simulink model "VFA_ActModel2_2015a"  (R2015a)
settings: Solver=ode23tb  SolverMode=SingleTasking  StartTime=tstart  StopTime=tsim  FixedStep=0.001  RelTol=1e-3
values from neighbouring files (symbols this model uses):
  Aa_M = zeros([10,10,length(TP.etasweep)])    [SimVFA.m]
  Ba32_aug_M = zeros([12,3,length(TP.etasweep)])    [SimVFA.m]
  Ba32_M = zeros([12,2,length(TP.etasweep)])    [SimVFA.m]
  Ba3_aug_M = zeros([12,3,length(TP.etasweep)])    [SimVFA.m]
  Ba3_M = zeros([12,2,length(TP.etasweep)])    [SimVFA.m]
  Ba_M = zeros([10,2,length(TP.etasweep)])    [SimVFA.m]
  Bp = TP.B_hold(:,1:5,SO.eta_nom+1)    [SimVFA.m]
  Ca = [C, zeros(size(C,1),length(index_output)) ... (first row only)    [SimVFA.m]
  Caz_M = zeros([2,10,length(TP.etasweep)])    [SimVFA.m]
  Cz = [0,0,0,0,1,0,0,0 ... (first row only)    [SimVFA.m]
  K_M = zeros([2,10,length(TP.etasweep)])    [SimVFA.m]
  L_M = zeros([10,3,length(TP.etasweep)])    [SimVFA.m]
  Rinv_M = zeros([3,3,length(TP.etasweep)])    [SimVFA.m]
  S1_M = zeros([2,3,length(TP.etasweep)])    [SimVFA.m]
  S_M = zeros([3,3,length(TP.etasweep)])    [SimVFA.m]
undefined symbols (not defined in the file or in its folder): a20, a21, a22, Aact, Acmd, Ada_Flag, ahold, Bact, Bact_x, Baz, Bcmd, Cact, Cact_dot, Ccmd, Ccmd_dot, cmd_filter_0, d00, d10, d11, d20, d21, d22, d_sam, data, Gamma_l, Gamma_p1, Gamma_p2, Gamma_p3, Gamma_p31, Gamma_p31xm, Gamma_p32, Gamma_vl, i_input_sel, i_state_sel, initstate, input_hold, inputselect, lambda_0, Lambda_s, mu_lambda, mu_psi1, mu_psi2, mu_psi3, mu_psi31, mu_psi32, n_sam, psi1_0, psi2_0, psi31_0, psi31xm_0, psi32_0, psi3_0, samplet, Si1, Si3, state_hold, vlambda_0, xact_0, xm_0
libraries: simulink x9
(part 2 of 2)

== system VFA_ActModel2_2015a/Adaptive Control/Fxm_Calculation/Filter13 ==
  u1 : Inport
  u1dot : Inport  Port=2
  u2 : Inport  Port=3
  u2dot : Inport  Port=4
  Gain2 : Gain  Gain=d10
  Gain25 : Gain  Gain=d11
  Matrix Multiply2 : Product  Multiplication=Matrix(*)
  Matrix Multiply3 : Product  Multiplication=Matrix(*)
  Sum2 : Sum  Inputs=++|
  Out1 : Outport
  wires:
  Matrix Multiply2/1 -> Gain2/1
  Matrix Multiply3/1 -> Gain25/1
  Gain25/1 -> Sum2/1
  u1dot/1 -> Matrix Multiply3/1
  u2/1 -> Matrix Multiply3/2
  u1/1 -> Matrix Multiply2/1
  u2dot/1 -> Matrix Multiply2/2
  Gain2/1 -> Sum2/2
  Sum2/1 -> Out1/1

== system VFA_ActModel2_2015a/Adaptive Control/Fxm_Calculation/Filter2 ==
  u1 : Inport
  u1dot : Inport  Port=2
  u2 : Inport  Port=3
  u2dot : Inport  Port=4
  Gain2 : Gain  Gain=d10
  Gain25 : Gain  Gain=d11
  Matrix Multiply2 : Product  Multiplication=Matrix(*)
  Matrix Multiply3 : Product  Multiplication=Matrix(*)
  Sum2 : Sum  Inputs=++|
  Out1 : Outport
  wires:
  Matrix Multiply2/1 -> Gain2/1
  Matrix Multiply3/1 -> Gain25/1
  Gain25/1 -> Sum2/1
  u1dot/1 -> Matrix Multiply3/1
  u2/1 -> Matrix Multiply3/2
  u1/1 -> Matrix Multiply2/1
  u2dot/1 -> Matrix Multiply2/2
  Gain2/1 -> Sum2/2
  Sum2/1 -> Out1/1

== system VFA_ActModel2_2015a/Adaptive Control/Fxm_Calculation/Filter3 ==
  u1 : Inport
  u1dot : Inport  Port=2
  u1ddot : Inport  Port=3
  u2 : Inport  Port=4
  u2dot : Inport  Port=5
  u2ddot : Inport  Port=6
  eta : Inport  Port=7
  Ba3 Interpolation : Subsystem
  Filter1 : Subsystem
      mask Display: disp('pi22 Mixer')
  Out1 : Outport
  wires:
  u2/1 -> Filter1/4(u2)
  u1/1 -> Filter1/1(u1)
  u1dot/1 -> Filter1/2(u1dot)
  u1ddot/1 -> Filter1/3(u1ddot)
  u2dot/1 -> Filter1/5(u2dot)
  u2ddot/1 -> Filter1/6(u2ddot)
  Filter1/1(Out1) -> Ba3 Interpolation/1(State)
  Ba3 Interpolation/1(Out1) -> Out1/1
  eta/1 -> Ba3 Interpolation/2(eta)

== system VFA_ActModel2_2015a/Adaptive Control/Fxm_Calculation/Filter4 ==
  In1 : Inport
  Add : Sum  Inputs=+--
  Add1 : Sum
  Add2 : Sum
  Gain1 : Gain  Gain=a21/a22
  Gain10 : Gain  Gain=1/a22
  Gain2 : Gain  Gain=a20/a22
  Gain3 : Gain  Gain=a21
  Gain4 : Gain  Gain=a21
  Gain{5..9} (5 alike) : Gain  Gain=a22
  Integrator : Integrator
  Integrator1 : Integrator
  pi20 filter : Outport
  pi20 filter dot : Outport  Port=2
  pi20 filter ddot : Outport  Port=3
  pi21 filter : Outport  Port=4
  pi21 filter dot : Outport  Port=5
  wires:
  Integrator/1 -> Gain1/1, Gain6/1, Integrator1/1, Gain4/1, Gain9/1  "out_dot"
  Add/1 -> Integrator/1, Gain8/1, Gain7/1  "out_ddot"
  Gain1/1 -> Add/3
  Gain2/1 -> Add/2
  Integrator1/1 -> Gain5/1, Gain3/1, Gain2/1  "out"
  Add1/1 -> pi21 filter/1
  Gain3/1 -> Add1/1
  Gain4/1 -> Add2/1
  Add2/1 -> pi21 filter dot/1
  Gain5/1 -> pi20 filter/1
  Gain6/1 -> pi20 filter dot/1
  Gain7/1 -> pi20 filter ddot/1
  Gain8/1 -> Add2/2
  Gain9/1 -> Add1/2
  In1/1 -> Gain10/1
  Gain10/1 -> Add/1

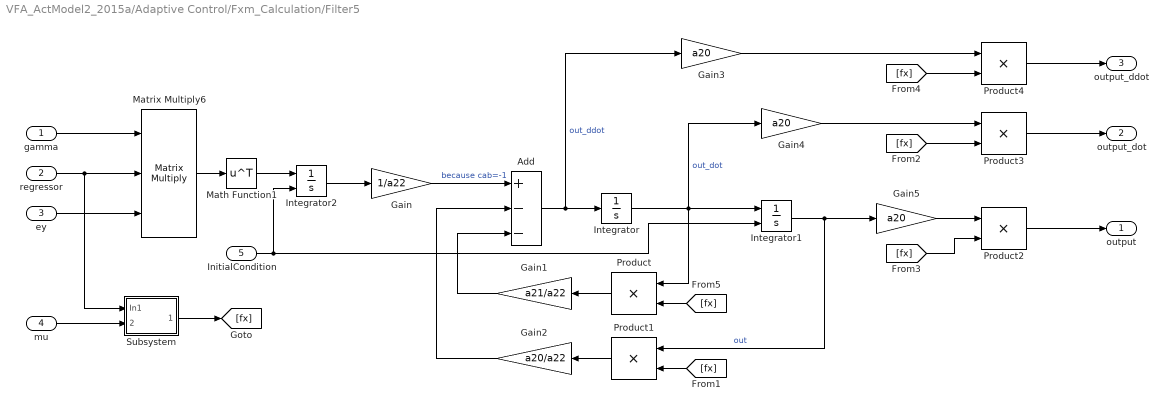
== system VFA_ActModel2_2015a/Adaptive Control/Fxm_Calculation/Filter5 ==
  gamma : Inport
  regressor : Inport  Port=2
  ey : Inport  Port=3
  mu : Inport  Port=4
  InitialCondition : Inport  Port=5
  Add : Sum  Inputs=+--
  Gain : Gain  Gain=1/a22
  Gain1 : Gain  Gain=a21/a22
  Gain2 : Gain  Gain=a20/a22
  Gain3 : Gain  Gain=a20
  Gain4 : Gain  Gain=a20
  Gain5 : Gain  Gain=a20
  Integrator : Integrator
  Integrator1 : Integrator  InitialConditionSource=external  InitialCondition=lambda_0'
  Integrator2 : Integrator  InitialConditionSource=external  InitialCondition=lambda_0'
  Math Function1 : Math  Operator=transpose  SaturateOnIntegerOverflow=on
  Matrix Multiply6 : Product  Inputs=3  Multiplication=Matrix(*)
  Product{,1..4} (5 alike) : Product  RndMeth=Zero
  Subsystem : Subsystem
      mask Display: disp('f(x)');
  output : Outport
  output_dot : Outport  Port=2
  output_ddot : Outport  Port=3
  wires:
  Integrator/1 -> Product/1, Gain4/1, Integrator1/1  "out_dot"
  Add/1 -> Integrator/1, Gain3/1  "out_ddot"
  Gain/1 -> Add/1  "because cab=-1"
  Gain1/1 -> Add/3
  Gain2/1 -> Add/2
  Integrator1/1 -> Product1/1, Gain5/1  "out"
  gamma/1 -> Matrix Multiply6/1
  regressor/1 -> Subsystem/1(In1), Matrix Multiply6/2
  ey/1 -> Matrix Multiply6/3
  Subsystem/1(Out1) -> [fx]
  Product/1 -> Gain1/1
  [fx] -> Product/2
  Product1/1 -> Gain2/1
  [fx] -> Product1/2
  Integrator2/1 -> Gain/1
  Gain5/1 -> Product2/1
  [fx] -> Product2/2
  Product2/1 -> output/1
  Gain4/1 -> Product3/1
  Product3/1 -> output_dot/1
  [fx] -> Product3/2
  [fx] -> Product4/2
  Gain3/1 -> Product4/1
  Product4/1 -> output_ddot/1
  Matrix Multiply6/1 -> Math Function1/1
  Math Function1/1 -> Integrator2/1
  InitialCondition/1 -> Integrator2/2, Integrator1/2
  mu/1 -> Subsystem/2(mu_psi)

== system VFA_ActModel2_2015a/Adaptive Control/Rinv and S Interpolation/Subsystem1 ==
  In1 : Inport
  In2 : Inport  Port=2
  Bias1 : Bias  Bias=1
  Direct Lookup Table (n-D)2 : LookupNDDirect  NumberOfTableDimensions=3  InputsSelectThisObjectFromTable=2-D Matrix  TableIsInput=on  Table=ahold
  Direct Lookup Table (n-D)3 : LookupNDDirect  NumberOfTableDimensions=3  InputsSelectThisObjectFromTable=2-D Matrix  TableIsInput=on  Table=ahold
  Fcn1 : Fcn  Expr=1-u(1)
  Prelookup1 : PreLookup  BreakpointsData=etasweep  ExtrapMethod=Linear
  Product2 : Product  RndMeth=Zero
  Product3 : Product  RndMeth=Zero
  Sum1 : Sum  Inputs=|++
  Out1 : Outport
  wires:
  In1/1 -> Prelookup1/1
  Sum1/1 -> Out1/1
  Prelookup1/1 -> Direct Lookup Table (n-D)3/1, Bias1/1
  Direct Lookup Table (n-D)2/1 -> Product2/1
  Prelookup1/2 -> Product2/2, Fcn1/1
  Direct Lookup Table (n-D)3/1 -> Product3/1
  Product2/1 -> Sum1/1
  Product3/1 -> Sum1/2
  Bias1/1 -> Direct Lookup Table (n-D)2/1
  In2/1 -> Direct Lookup Table (n-D)3/2, Direct Lookup Table (n-D)2/2
  Fcn1/1 -> Product3/2

== system VFA_ActModel2_2015a/Adaptive Control/Rinv and S Interpolation/Subsystem2 ==
  In1 : Inport
  In2 : Inport  Port=2
  Bias1 : Bias  Bias=1
  Direct Lookup Table (n-D)2 : LookupNDDirect  NumberOfTableDimensions=3  InputsSelectThisObjectFromTable=2-D Matrix  TableIsInput=on  Table=ahold
  Direct Lookup Table (n-D)3 : LookupNDDirect  NumberOfTableDimensions=3  InputsSelectThisObjectFromTable=2-D Matrix  TableIsInput=on  Table=ahold
  Fcn1 : Fcn  Expr=1-u(1)
  Prelookup1 : PreLookup  BreakpointsData=etasweep  ExtrapMethod=Linear
  Product2 : Product  RndMeth=Zero
  Product3 : Product  RndMeth=Zero
  Sum1 : Sum  Inputs=|++
  Out1 : Outport
  wires:
  In1/1 -> Prelookup1/1
  Sum1/1 -> Out1/1
  Prelookup1/1 -> Direct Lookup Table (n-D)3/1, Bias1/1
  Direct Lookup Table (n-D)2/1 -> Product2/1
  Prelookup1/2 -> Product2/2, Fcn1/1
  Direct Lookup Table (n-D)3/1 -> Product3/1
  Product2/1 -> Sum1/1
  Product3/1 -> Sum1/2
  Bias1/1 -> Direct Lookup Table (n-D)2/1
  In2/1 -> Direct Lookup Table (n-D)3/2, Direct Lookup Table (n-D)2/2
  Fcn1/1 -> Product3/2

== system VFA_ActModel2_2015a/Adaptive Control/S Interpolation/Subsystem1 ==
  In1 : Inport
  In2 : Inport  Port=2
  Bias1 : Bias  Bias=1
  Direct Lookup Table (n-D)2 : LookupNDDirect  NumberOfTableDimensions=3  InputsSelectThisObjectFromTable=2-D Matrix  TableIsInput=on  Table=ahold
  Direct Lookup Table (n-D)3 : LookupNDDirect  NumberOfTableDimensions=3  InputsSelectThisObjectFromTable=2-D Matrix  TableIsInput=on  Table=ahold
  Fcn1 : Fcn  Expr=1-u(1)
  Prelookup1 : PreLookup  BreakpointsData=etasweep  ExtrapMethod=Linear
  Product2 : Product  RndMeth=Zero
  Product3 : Product  RndMeth=Zero
  Sum1 : Sum  Inputs=|++
  Out1 : Outport
  wires:
  In1/1 -> Prelookup1/1
  Sum1/1 -> Out1/1
  Prelookup1/1 -> Direct Lookup Table (n-D)3/1, Bias1/1
  Direct Lookup Table (n-D)2/1 -> Product2/1
  Prelookup1/2 -> Product2/2, Fcn1/1
  Direct Lookup Table (n-D)3/1 -> Product3/1
  Product2/1 -> Sum1/1
  Product3/1 -> Sum1/2
  Bias1/1 -> Direct Lookup Table (n-D)2/1
  In2/1 -> Direct Lookup Table (n-D)3/2, Direct Lookup Table (n-D)2/2
  Fcn1/1 -> Product3/2

== system VFA_ActModel2_2015a/Adaptive Control/S1 Interpolation/Subsystem1 ==
  In1 : Inport
  In2 : Inport  Port=2
  Bias1 : Bias  Bias=1
  Direct Lookup Table (n-D)2 : LookupNDDirect  NumberOfTableDimensions=3  InputsSelectThisObjectFromTable=2-D Matrix  TableIsInput=on  Table=ahold
  Direct Lookup Table (n-D)3 : LookupNDDirect  NumberOfTableDimensions=3  InputsSelectThisObjectFromTable=2-D Matrix  TableIsInput=on  Table=ahold
  Fcn1 : Fcn  Expr=1-u(1)
  Prelookup1 : PreLookup  BreakpointsData=etasweep  ExtrapMethod=Linear
  Product2 : Product  RndMeth=Zero
  Product3 : Product  RndMeth=Zero
  Sum1 : Sum  Inputs=|++
  Out1 : Outport
  wires:
  In1/1 -> Prelookup1/1
  Sum1/1 -> Out1/1
  Prelookup1/1 -> Direct Lookup Table (n-D)3/1, Bias1/1
  Direct Lookup Table (n-D)2/1 -> Product2/1
  Prelookup1/2 -> Product2/2, Fcn1/1
  Direct Lookup Table (n-D)3/1 -> Product3/1
  Product2/1 -> Sum1/1
  Product3/1 -> Sum1/2
  Bias1/1 -> Direct Lookup Table (n-D)2/1
  In2/1 -> Direct Lookup Table (n-D)3/2, Direct Lookup Table (n-D)2/2
  Fcn1/1 -> Product3/2

== system VFA_ActModel2_2015a/Adaptive Control/uad_Calculation/Filter1 ==
  u1 : Inport
  u1dot : Inport  Port=2
  u1ddot : Inport  Port=3
  u2 : Inport  Port=4
  u2dot : Inport  Port=5
  u2ddot : Inport  Port=6
  Gain1 : Gain  Gain=d21
  Gain2 : Gain  Gain=d20
  Gain3 : Gain  Gain=d22
  Gain4 : Gain  Gain=a22
  Gain5 : Gain  Gain=d11
  Gain6 : Gain  Gain=d10
  Gain7 : Gain  Gain=a21
  Gain8 : Gain  Gain=d00
  Gain9 : Gain  Gain=a20
  Matrix Multiply{1..6} (6 alike) : Product  Multiplication=Matrix(*)
  Sum1 : Sum  Inputs=+++|
  Sum2 : Sum  Inputs=+++|
  Sum3 : Sum  Inputs=++|
  Out1 : Outport
  wires:
  u1/1 -> Matrix Multiply2/1, Matrix Multiply6/1, Matrix Multiply5/1
  u2ddot/1 -> Matrix Multiply2/2
  Matrix Multiply2/1 -> Gain2/1
  u1ddot/1 -> Matrix Multiply1/1
  u2/1 -> Matrix Multiply6/2, Matrix Multiply4/2, Matrix Multiply1/2
  Matrix Multiply1/1 -> Gain3/1
  u2dot/1 -> Matrix Multiply5/2, Matrix Multiply3/2
  u1dot/1 -> Matrix Multiply4/1, Matrix Multiply3/1
  Matrix Multiply3/1 -> Gain1/1
  Gain1/1 -> Sum1/3
  Gain3/1 -> Sum1/2
  Gain2/1 -> Sum1/1
  Sum1/1 -> Gain4/1
  Gain4/1 -> Sum2/1
  Matrix Multiply4/1 -> Gain5/1
  Gain5/1 -> Sum3/1
  Matrix Multiply5/1 -> Gain6/1
  Gain6/1 -> Sum3/2
  Sum3/1 -> Gain7/1
  Gain7/1 -> Sum2/2
  Matrix Multiply6/1 -> Gain8/1
  Gain8/1 -> Gain9/1
  Sum2/1 -> Out1/1
  Gain9/1 -> Sum2/3

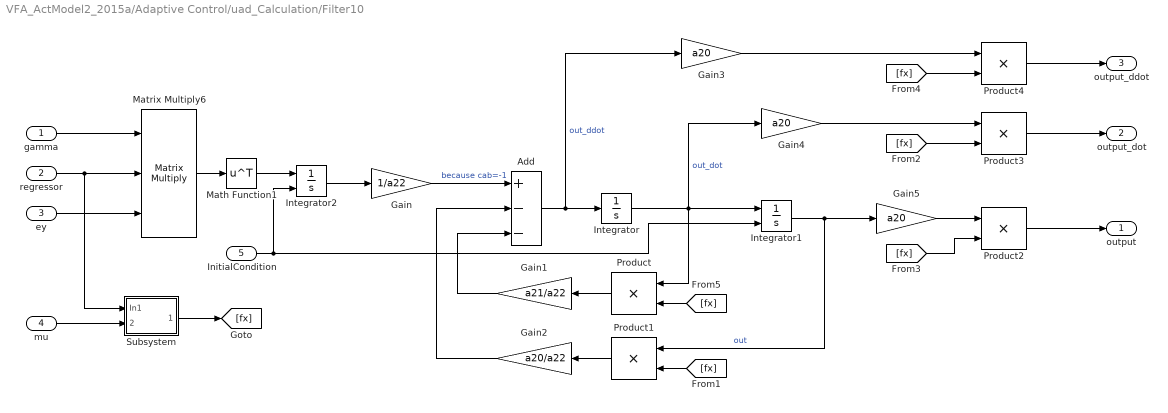
== system VFA_ActModel2_2015a/Adaptive Control/uad_Calculation/Filter10 ==
  gamma : Inport
  regressor : Inport  Port=2
  ey : Inport  Port=3
  mu : Inport  Port=4
  InitialCondition : Inport  Port=5
  Add : Sum  Inputs=+--
  Gain : Gain  Gain=1/a22
  Gain1 : Gain  Gain=a21/a22
  Gain2 : Gain  Gain=a20/a22
  Gain3 : Gain  Gain=a20
  Gain4 : Gain  Gain=a20
  Gain5 : Gain  Gain=a20
  Integrator : Integrator
  Integrator1 : Integrator  InitialConditionSource=external  InitialCondition=lambda_0'
  Integrator2 : Integrator  InitialConditionSource=external  InitialCondition=lambda_0'
  Math Function1 : Math  Operator=transpose  SaturateOnIntegerOverflow=on
  Matrix Multiply6 : Product  Inputs=3  Multiplication=Matrix(*)
  Product{,1..4} (5 alike) : Product  RndMeth=Zero
  Subsystem : Subsystem
      mask Display: disp('f(x)');
  output : Outport
  output_dot : Outport  Port=2
  output_ddot : Outport  Port=3
  wires:
  Integrator/1 -> Product/1, Gain4/1, Integrator1/1  "out_dot"
  Add/1 -> Integrator/1, Gain3/1  "out_ddot"
  Gain/1 -> Add/1  "because cab=-1"
  Gain1/1 -> Add/3
  Gain2/1 -> Add/2
  Integrator1/1 -> Product1/1, Gain5/1  "out"
  gamma/1 -> Matrix Multiply6/1
  regressor/1 -> Subsystem/1(In1), Matrix Multiply6/2
  ey/1 -> Matrix Multiply6/3
  Subsystem/1(Out1) -> [fx]
  Product/1 -> Gain1/1
  [fx] -> Product/2
  Product1/1 -> Gain2/1
  [fx] -> Product1/2
  Integrator2/1 -> Gain/1
  Gain5/1 -> Product2/1
  [fx] -> Product2/2
  Product2/1 -> output/1
  Gain4/1 -> Product3/1
  Product3/1 -> output_dot/1
  [fx] -> Product3/2
  [fx] -> Product4/2
  Gain3/1 -> Product4/1
  Product4/1 -> output_ddot/1
  Matrix Multiply6/1 -> Math Function1/1
  Math Function1/1 -> Integrator2/1
  InitialCondition/1 -> Integrator2/2, Integrator1/2
  mu/1 -> Subsystem/2(mu_psi)

== system VFA_ActModel2_2015a/Adaptive Control/uad_Calculation/Filter11 ==
  u1 : Inport
  u1dot : Inport  Port=2
  u1ddot : Inport  Port=3
  u2 : Inport  Port=4
  u2dot : Inport  Port=5
  u2ddot : Inport  Port=6
  Gain1 : Gain  Gain=d21
  Gain2 : Gain  Gain=d20
  Gain3 : Gain  Gain=d22
  Gain4 : Gain  Gain=a22
  Gain5 : Gain  Gain=d11
  Gain6 : Gain  Gain=d10
  Gain7 : Gain  Gain=a21
  Gain8 : Gain  Gain=d00
  Gain9 : Gain  Gain=a20
  Matrix Multiply{1..6} (6 alike) : Product  Multiplication=Matrix(*)
  Sum1 : Sum  Inputs=+++|
  Sum2 : Sum  Inputs=+++|
  Sum3 : Sum  Inputs=++|
  Out1 : Outport
  wires:
  u1/1 -> Matrix Multiply2/1, Matrix Multiply6/1, Matrix Multiply5/1
  u2ddot/1 -> Matrix Multiply2/2
  Matrix Multiply2/1 -> Gain2/1
  u1ddot/1 -> Matrix Multiply1/1
  u2/1 -> Matrix Multiply6/2, Matrix Multiply4/2, Matrix Multiply1/2
  Matrix Multiply1/1 -> Gain3/1
  u2dot/1 -> Matrix Multiply5/2, Matrix Multiply3/2
  u1dot/1 -> Matrix Multiply4/1, Matrix Multiply3/1
  Matrix Multiply3/1 -> Gain1/1
  Gain1/1 -> Sum1/3
  Gain3/1 -> Sum1/2
  Gain2/1 -> Sum1/1
  Sum1/1 -> Gain4/1
  Gain4/1 -> Sum2/1
  Matrix Multiply4/1 -> Gain5/1
  Gain5/1 -> Sum3/1
  Matrix Multiply5/1 -> Gain6/1
  Gain6/1 -> Sum3/2
  Sum3/1 -> Gain7/1
  Gain7/1 -> Sum2/2
  Matrix Multiply6/1 -> Gain8/1
  Gain8/1 -> Gain9/1
  Sum2/1 -> Out1/1
  Gain9/1 -> Sum2/3

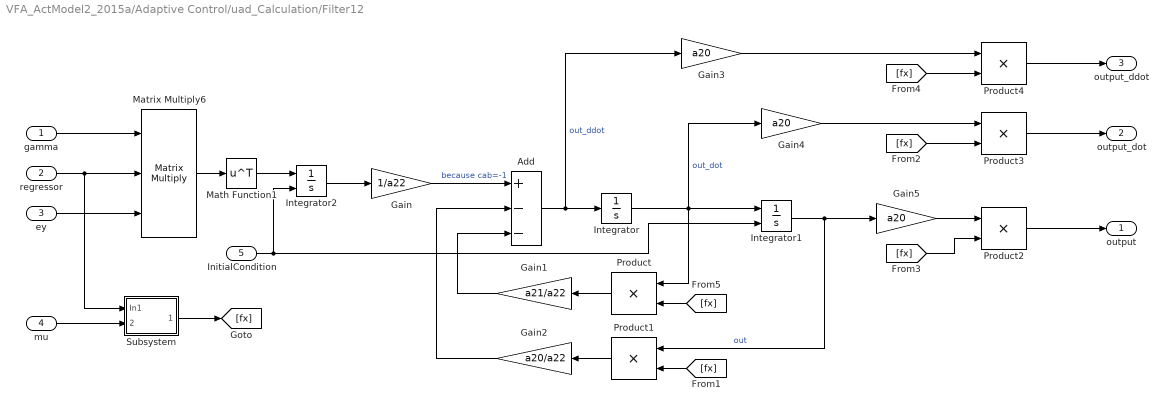
== system VFA_ActModel2_2015a/Adaptive Control/uad_Calculation/Filter12 ==
  gamma : Inport
  regressor : Inport  Port=2
  ey : Inport  Port=3
  mu : Inport  Port=4
  InitialCondition : Inport  Port=5
  Add : Sum  Inputs=+--
  Gain : Gain  Gain=1/a22
  Gain1 : Gain  Gain=a21/a22
  Gain2 : Gain  Gain=a20/a22
  Gain3 : Gain  Gain=a20
  Gain4 : Gain  Gain=a20
  Gain5 : Gain  Gain=a20
  Integrator : Integrator
  Integrator1 : Integrator  InitialConditionSource=external  InitialCondition=lambda_0'
  Integrator2 : Integrator  InitialConditionSource=external  InitialCondition=lambda_0'
  Math Function1 : Math  Operator=transpose  SaturateOnIntegerOverflow=on
  Matrix Multiply6 : Product  Inputs=3  Multiplication=Matrix(*)
  Product{,1..4} (5 alike) : Product  RndMeth=Zero
  Subsystem : Subsystem
      mask Display: disp('f(x)');
  output : Outport
  output_dot : Outport  Port=2
  output_ddot : Outport  Port=3
  wires:
  Integrator/1 -> Product/1, Gain4/1, Integrator1/1  "out_dot"
  Add/1 -> Integrator/1, Gain3/1  "out_ddot"
  Gain/1 -> Add/1  "because cab=-1"
  Gain1/1 -> Add/3
  Gain2/1 -> Add/2
  Integrator1/1 -> Product1/1, Gain5/1  "out"
  gamma/1 -> Matrix Multiply6/1
  regressor/1 -> Subsystem/1(In1), Matrix Multiply6/2
  ey/1 -> Matrix Multiply6/3
  Subsystem/1(Out1) -> [fx]
  Product/1 -> Gain1/1
  [fx] -> Product/2
  Product1/1 -> Gain2/1
  [fx] -> Product1/2
  Integrator2/1 -> Gain/1
  Gain5/1 -> Product2/1
  [fx] -> Product2/2
  Product2/1 -> output/1
  Gain4/1 -> Product3/1
  Product3/1 -> output_dot/1
  [fx] -> Product3/2
  [fx] -> Product4/2
  Gain3/1 -> Product4/1
  Product4/1 -> output_ddot/1
  Matrix Multiply6/1 -> Math Function1/1
  Math Function1/1 -> Integrator2/1
  InitialCondition/1 -> Integrator2/2, Integrator1/2
  mu/1 -> Subsystem/2(mu_psi)

== system VFA_ActModel2_2015a/Adaptive Control/uad_Calculation/Filter13 ==
  In1 : Inport
  In1_dot : Inport  Port=2
  Add : Sum  Inputs=+--
  Add1 : Sum
  Add2 : Sum
  Add3 : Sum  Inputs=-+
  Gain1 : Gain  Gain=a21/a22
  Gain10 : Gain  Gain=1/a22
  Gain11 : Gain  Gain=a20
  Gain2 : Gain  Gain=a20/a22
  Gain3 : Gain  Gain=a21
  Gain4 : Gain  Gain=a21
  Gain{5..9} (5 alike) : Gain  Gain=a22
  Integrator : Integrator
  Integrator1 : Integrator
  pi20 filter : Outport
  pi20 filter dot : Outport  Port=2
  pi20 filter ddot : Outport  Port=3
  pi21 filter : Outport  Port=4
  pi21 filter dot : Outport  Port=5
  pi21 filter ddot : Outport  Port=6
  wires:
  Integrator/1 -> Gain1/1, Gain11/1, Gain4/1, Gain9/1, Integrator1/1, Gain6/1  "out_dot"
  Add/1 -> Integrator/1, Gain8/1, Gain7/1  "out_ddot"
  Gain1/1 -> Add/3
  Gain2/1 -> Add/2
  Integrator1/1 -> Gain5/1, Gain3/1, Gain2/1  "out"
  Add1/1 -> pi21 filter/1
  Gain3/1 -> Add1/1
  Gain4/1 -> Add2/1
  Add2/1 -> pi21 filter dot/1
  Gain5/1 -> pi20 filter/1
  Gain6/1 -> pi20 filter dot/1
  Gain7/1 -> pi20 filter ddot/1
  Gain8/1 -> Add2/2
  Gain9/1 -> Add1/2
  In1/1 -> Gain10/1
  Gain10/1 -> Add/1
  Add3/1 -> pi21 filter ddot/1
  In1_dot/1 -> Add3/2
  Gain11/1 -> Add3/1

== system VFA_ActModel2_2015a/Adaptive Control/uad_Calculation/Filter2 ==
  u1 : Inport
  u1dot : Inport  Port=2
  u1ddot : Inport  Port=3
  u2 : Inport  Port=4
  u2dot : Inport  Port=5
  u2ddot : Inport  Port=6
  Gain1 : Gain  Gain=d21
  Gain2 : Gain  Gain=d20
  Gain3 : Gain  Gain=d22
  Gain4 : Gain  Gain=a22
  Gain5 : Gain  Gain=d11
  Gain6 : Gain  Gain=d10
  Gain7 : Gain  Gain=a21
  Gain8 : Gain  Gain=d00
  Gain9 : Gain  Gain=a20
  Matrix Multiply{1..6} (6 alike) : Product  Multiplication=Matrix(*)
  Sum1 : Sum  Inputs=+++|
  Sum2 : Sum  Inputs=+++|
  Sum3 : Sum  Inputs=++|
  Out1 : Outport
  wires:
  u1/1 -> Matrix Multiply2/1, Matrix Multiply6/1, Matrix Multiply5/1
  u2ddot/1 -> Matrix Multiply2/2
  Matrix Multiply2/1 -> Gain2/1
  u1ddot/1 -> Matrix Multiply1/1
  u2/1 -> Matrix Multiply6/2, Matrix Multiply4/2, Matrix Multiply1/2
  Matrix Multiply1/1 -> Gain3/1
  u2dot/1 -> Matrix Multiply5/2, Matrix Multiply3/2
  u1dot/1 -> Matrix Multiply4/1, Matrix Multiply3/1
  Matrix Multiply3/1 -> Gain1/1
  Gain1/1 -> Sum1/3
  Gain3/1 -> Sum1/2
  Gain2/1 -> Sum1/1
  Sum1/1 -> Gain4/1
  Gain4/1 -> Sum2/1
  Matrix Multiply4/1 -> Gain5/1
  Gain5/1 -> Sum3/1
  Matrix Multiply5/1 -> Gain6/1
  Gain6/1 -> Sum3/2
  Sum3/1 -> Gain7/1
  Gain7/1 -> Sum2/2
  Matrix Multiply6/1 -> Gain8/1
  Gain8/1 -> Gain9/1
  Sum2/1 -> Out1/1
  Gain9/1 -> Sum2/3

== system VFA_ActModel2_2015a/Adaptive Control/uad_Calculation/Filter3 ==
  u1 : Inport
  u1dot : Inport  Port=2
  u1ddot : Inport  Port=3
  u2 : Inport  Port=4
  u2dot : Inport  Port=5
  u2ddot : Inport  Port=6
  Gain1 : Gain  Gain=d21
  Gain2 : Gain  Gain=d20
  Gain3 : Gain  Gain=d22
  Gain4 : Gain  Gain=a22
  Gain5 : Gain  Gain=d11
  Gain6 : Gain  Gain=d10
  Gain7 : Gain  Gain=a21
  Gain8 : Gain  Gain=d00
  Gain9 : Gain  Gain=a20
  Matrix Multiply{1..6} (6 alike) : Product  Multiplication=Matrix(*)
  Sum1 : Sum  Inputs=+++|
  Sum2 : Sum  Inputs=+++|
  Sum3 : Sum  Inputs=++|
  Out1 : Outport
  wires:
  u1/1 -> Matrix Multiply2/1, Matrix Multiply6/1, Matrix Multiply5/1
  u2ddot/1 -> Matrix Multiply2/2
  Matrix Multiply2/1 -> Gain2/1
  u1ddot/1 -> Matrix Multiply1/1
  u2/1 -> Matrix Multiply6/2, Matrix Multiply4/2, Matrix Multiply1/2
  Matrix Multiply1/1 -> Gain3/1
  u2dot/1 -> Matrix Multiply5/2, Matrix Multiply3/2
  u1dot/1 -> Matrix Multiply4/1, Matrix Multiply3/1
  Matrix Multiply3/1 -> Gain1/1
  Gain1/1 -> Sum1/3
  Gain3/1 -> Sum1/2
  Gain2/1 -> Sum1/1
  Sum1/1 -> Gain4/1
  Gain4/1 -> Sum2/1
  Matrix Multiply4/1 -> Gain5/1
  Gain5/1 -> Sum3/1
  Matrix Multiply5/1 -> Gain6/1
  Gain6/1 -> Sum3/2
  Sum3/1 -> Gain7/1
  Gain7/1 -> Sum2/2
  Matrix Multiply6/1 -> Gain8/1
  Gain8/1 -> Gain9/1
  Sum2/1 -> Out1/1
  Gain9/1 -> Sum2/3

== system VFA_ActModel2_2015a/Adaptive Control/uad_Calculation/Filter4 ==
  note: out_ddot
  In1 : Inport
  Gain : Gain  Gain=1/a22
  Gain1 : Gain  Gain=a21/a22
  Gain2 : Gain  Gain=a20/a22
  Integrator : Integrator
  Integrator1 : Integrator
  Sum : Sum  Inputs=|+--
  Out1 : Outport
  Out2 : Outport  Port=2
  Out3 : Outport  Port=3
  wires:
  In1/1 -> Gain/1
  Gain/1 -> Sum/1
  Gain1/1 -> Sum/3
  Gain2/1 -> Sum/2
  Integrator1/1 -> Out1/1, Gain2/1  "out"
  Integrator/1 -> Gain1/1, Out2/1, Integrator1/1  "out_dot"
  Sum/1 -> Out3/1, Integrator/1

== system VFA_ActModel2_2015a/Adaptive Control/uad_Calculation/Filter5 ==
  xm : Inport
  r : Inport  Port=2
  r_dot : Inport  Port=3
  ey : Inport  Port=4
  Add : Sum  Inputs=2
  Add1 : Sum  Inputs=+++-
  Gain1 : Gain  Gain=Baz  Multiplication=Matrix(K*u)
  Gain2 : Gain  Gain=Baz  Multiplication=Matrix(K*u)
  Gain4 : Gain  Gain=Baz  Multiplication=Matrix(K*u)
  Matrix Multiply1 : Product  Inputs=3  Multiplication=Matrix(*)
  Matrix Multiply2 : Product  Multiplication=Matrix(*)
  Matrix Multiply3 : Product  Multiplication=Matrix(*)
  Matrix Multiply4 : Product  Inputs=3  Multiplication=Matrix(*)
  Out1 : Outport
  Out1_dot : Outport  Port=2
  Out1_ddot : Outport  Port=3
  wires:
  Matrix Multiply2/1 -> Add/1
  r/1 -> Gain2/1, Gain1/1
  r_dot/1 -> Gain4/1
  ey/1 -> Matrix Multiply4/3
  Add1/1 -> Out1_ddot/1  "(A^2)*xm + A*Bz*r + Bz*r_dot + A*L*ey"
  Gain1/1 -> Add/2
  Add/1 -> Out1_dot/1  "A*xm + Bz*r"
  Matrix Multiply1/1 -> Add1/1
  Matrix Multiply3/1 -> Add1/2
  Gain4/1 -> Add1/3
  Matrix Multiply4/1 -> Add1/4
  [Aa] -> Matrix Multiply2/1
  [Aa] -> Matrix Multiply1/1, Matrix Multiply1/2
  xm/1 -> Out1/1, Matrix Multiply1/3, Matrix Multiply2/2  "xm"
  [Aa] -> Matrix Multiply3/1
  [L] -> Matrix Multiply4/2
  [Aa] -> Matrix Multiply4/1
  Gain2/1 -> Matrix Multiply3/2

== system VFA_ActModel2_2015a/Adaptive Control/uad_Calculation/Filter6 ==
  In1 : Inport
  Integrator1 : Integrator
  Out1 : Outport
  Out1_dot : Outport  Port=2
  wires:
  Integrator1/1 -> Out1/1  "out"
  In1/1 -> Out1_dot/1, Integrator1/1

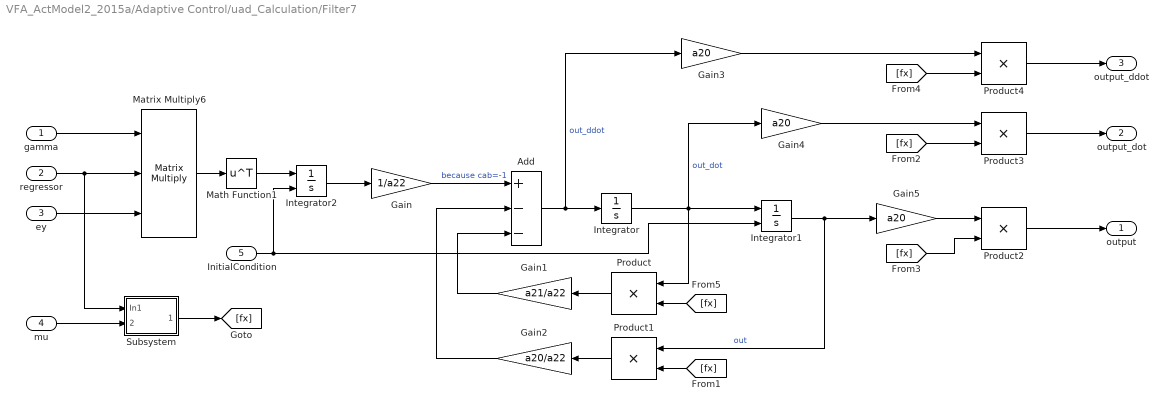
== system VFA_ActModel2_2015a/Adaptive Control/uad_Calculation/Filter7 ==
  gamma : Inport
  regressor : Inport  Port=2
  ey : Inport  Port=3
  mu : Inport  Port=4
  InitialCondition : Inport  Port=5
  Add : Sum  Inputs=+--
  Gain : Gain  Gain=1/a22
  Gain1 : Gain  Gain=a21/a22
  Gain2 : Gain  Gain=a20/a22
  Gain3 : Gain  Gain=a20
  Gain4 : Gain  Gain=a20
  Gain5 : Gain  Gain=a20
  Integrator : Integrator
  Integrator1 : Integrator  InitialConditionSource=external  InitialCondition=lambda_0'
  Integrator2 : Integrator  InitialConditionSource=external  InitialCondition=lambda_0'
  Math Function1 : Math  Operator=transpose  SaturateOnIntegerOverflow=on
  Matrix Multiply6 : Product  Inputs=3  Multiplication=Matrix(*)
  Product{,1..4} (5 alike) : Product  RndMeth=Zero
  Subsystem : Subsystem
      mask Display: disp('f(x)');
  output : Outport
  output_dot : Outport  Port=2
  output_ddot : Outport  Port=3
  wires:
  Integrator/1 -> Product/1, Gain4/1, Integrator1/1  "out_dot"
  Add/1 -> Integrator/1, Gain3/1  "out_ddot"
  Gain/1 -> Add/1  "because cab=-1"
  Gain1/1 -> Add/3
  Gain2/1 -> Add/2
  Integrator1/1 -> Product1/1, Gain5/1  "out"
  gamma/1 -> Matrix Multiply6/1
  regressor/1 -> Subsystem/1(In1), Matrix Multiply6/2
  ey/1 -> Matrix Multiply6/3
  Subsystem/1(Out1) -> [fx]
  Product/1 -> Gain1/1
  [fx] -> Product/2
  Product1/1 -> Gain2/1
  [fx] -> Product1/2
  Integrator2/1 -> Gain/1
  Gain5/1 -> Product2/1
  [fx] -> Product2/2
  Product2/1 -> output/1
  Gain4/1 -> Product3/1
  Product3/1 -> output_dot/1
  [fx] -> Product3/2
  [fx] -> Product4/2
  Gain3/1 -> Product4/1
  Product4/1 -> output_ddot/1
  Matrix Multiply6/1 -> Math Function1/1
  Math Function1/1 -> Integrator2/1
  InitialCondition/1 -> Integrator2/2, Integrator1/2
  mu/1 -> Subsystem/2(mu_psi)

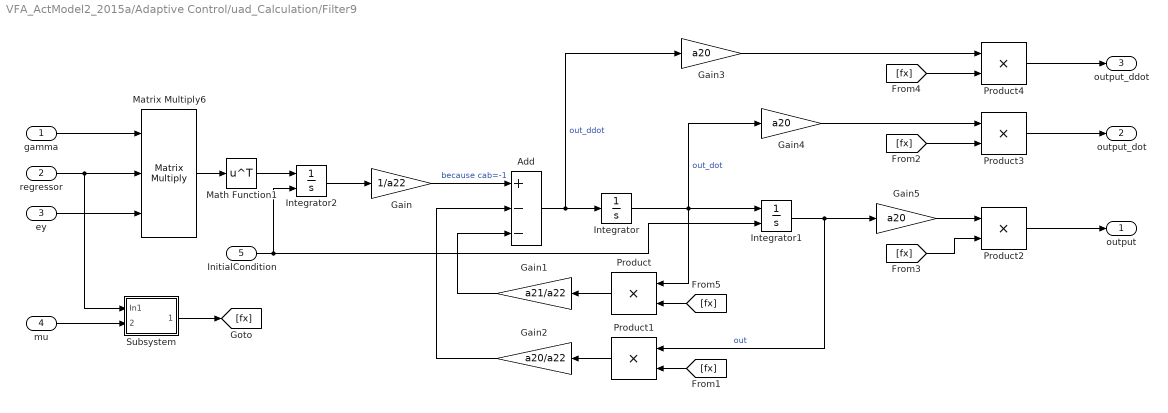
== system VFA_ActModel2_2015a/Adaptive Control/uad_Calculation/Filter9 ==
  gamma : Inport
  regressor : Inport  Port=2
  ey : Inport  Port=3
  mu : Inport  Port=4
  InitialCondition : Inport  Port=5
  Add : Sum  Inputs=+--
  Gain : Gain  Gain=1/a22
  Gain1 : Gain  Gain=a21/a22
  Gain2 : Gain  Gain=a20/a22
  Gain3 : Gain  Gain=a20
  Gain4 : Gain  Gain=a20
  Gain5 : Gain  Gain=a20
  Integrator : Integrator
  Integrator1 : Integrator  InitialConditionSource=external  InitialCondition=lambda_0'
  Integrator2 : Integrator  InitialConditionSource=external  InitialCondition=lambda_0'
  Math Function1 : Math  Operator=transpose  SaturateOnIntegerOverflow=on
  Matrix Multiply6 : Product  Inputs=3  Multiplication=Matrix(*)
  Product{,1..4} (5 alike) : Product  RndMeth=Zero
  Subsystem : Subsystem
      mask Display: disp('f(x)');
  output : Outport
  output_dot : Outport  Port=2
  output_ddot : Outport  Port=3
  wires:
  Integrator/1 -> Product/1, Gain4/1, Integrator1/1  "out_dot"
  Add/1 -> Integrator/1, Gain3/1  "out_ddot"
  Gain/1 -> Add/1  "because cab=-1"
  Gain1/1 -> Add/3
  Gain2/1 -> Add/2
  Integrator1/1 -> Product1/1, Gain5/1  "out"
  gamma/1 -> Matrix Multiply6/1
  regressor/1 -> Subsystem/1(In1), Matrix Multiply6/2
  ey/1 -> Matrix Multiply6/3
  Subsystem/1(Out1) -> [fx]
  Product/1 -> Gain1/1
  [fx] -> Product/2
  Product1/1 -> Gain2/1
  [fx] -> Product1/2
  Integrator2/1 -> Gain/1
  Gain5/1 -> Product2/1
  [fx] -> Product2/2
  Product2/1 -> output/1
  Gain4/1 -> Product3/1
  Product3/1 -> output_dot/1
  [fx] -> Product3/2
  [fx] -> Product4/2
  Gain3/1 -> Product4/1
  Product4/1 -> output_ddot/1
  Matrix Multiply6/1 -> Math Function1/1
  Math Function1/1 -> Integrator2/1
  InitialCondition/1 -> Integrator2/2, Integrator1/2
  mu/1 -> Subsystem/2(mu_psi)

== system VFA_ActModel2_2015a/Aircraft (Plant)/NonLinear VFA Model/Input Trim ==
  Constant1 : Constant  Value=[1:5]
  Constant2 : Constant  Value=input_hold
  Selector1 : Selector  InputPortWidth=9  IndexOptions=Index vector (port)  Indices=[1 3]  OutputSizes=1
  u_trim : Outport
  wires:
  Constant1/1 -> Selector1/2
  Constant2/1 -> Selector1/1
  Selector1/1 -> u_trim/1

== system VFA_ActModel2_2015a/Aircraft (Plant)/NonLinear VFA Model/State Trim ==
  Constant3 : Constant  Value=state_hold
  Constant5 : Constant  Value=i_state_sel
  Selector2 : Selector  InputPortWidth=length(Bp)  IndexOptions=Index vector (port)  Indices=[1 3]  OutputSizes=1
  To Workspace3 : ToWorkspace  VariableName=x_hold  SampleTime=-1
      settings: Decimation=data_deci
  x_trim : Outport
  wires:
  Constant5/1 -> Selector2/2
  Constant3/1 -> Selector2/1
  Selector2/1 -> To Workspace3/1, x_trim/1

== system VFA_ActModel2_2015a/Adaptive Control/FL_Calculation/Filter1/Ba32_aug Interpolation ==
  State : Inport
  eta : Inport  Port=2
  Constant2 : Constant  Value=Ba32_aug_M
  Gain : Gain  Gain=180/pi
  Matrix Multiply6 : Product  Multiplication=Matrix(*)
  Subsystem1 : Subsystem
      mask Display: disp('matrix-interp');
  Out1 : Outport
  wires:
  eta/1 -> Gain/1
  Gain/1 -> Subsystem1/1(In1)
  Subsystem1/1(Out1) -> Matrix Multiply6/1
  State/1 -> Matrix Multiply6/2
  Matrix Multiply6/1 -> Out1/1
  Constant2/1 -> Subsystem1/2(In2)

== system VFA_ActModel2_2015a/Adaptive Control/FL_Calculation/Filter1/Ba3_aug Interpolation ==
  State : Inport
  eta : Inport  Port=2
  Constant2 : Constant  Value=Ba3_aug_M
  Gain : Gain  Gain=180/pi
  Matrix Multiply6 : Product  Multiplication=Matrix(*)
  Subsystem1 : Subsystem
      mask Display: disp('matrix-interp');
  Out1 : Outport
  wires:
  eta/1 -> Gain/1
  Gain/1 -> Subsystem1/1(In1)
  Subsystem1/1(Out1) -> Matrix Multiply6/1
  State/1 -> Matrix Multiply6/2
  Matrix Multiply6/1 -> Out1/1
  Constant2/1 -> Subsystem1/2(In2)

== system VFA_ActModel2_2015a/Adaptive Control/FL_Calculation/Filter1/Filter15 ==
  u1 : Inport
  u1dot : Inport  Port=2
  u2 : Inport  Port=3
  u2dot : Inport  Port=4
  Gain2 : Gain  Gain=d10
  Gain25 : Gain  Gain=d11
  Matrix Multiply2 : Product  Multiplication=Matrix(*)
  Matrix Multiply3 : Product  Multiplication=Matrix(*)
  Sum2 : Sum  Inputs=++|
  Out1 : Outport
  wires:
  Matrix Multiply2/1 -> Gain2/1
  Matrix Multiply3/1 -> Gain25/1
  Gain25/1 -> Sum2/1
  u1dot/1 -> Matrix Multiply3/1
  u2/1 -> Matrix Multiply3/2
  u1/1 -> Matrix Multiply2/1
  u2dot/1 -> Matrix Multiply2/2
  Gain2/1 -> Sum2/2
  Sum2/1 -> Out1/1

== system VFA_ActModel2_2015a/Adaptive Control/FL_Calculation/Filter2/Ba3_aug Interpolation ==
  State : Inport
  eta : Inport  Port=2
  Constant2 : Constant  Value=Ba3_aug_M
  Gain : Gain  Gain=180/pi
  Matrix Multiply6 : Product  Multiplication=Matrix(*)
  Subsystem1 : Subsystem
      mask Display: disp('matrix-interp');
  Out1 : Outport
  wires:
  eta/1 -> Gain/1
  Gain/1 -> Subsystem1/1(In1)
  Subsystem1/1(Out1) -> Matrix Multiply6/1
  State/1 -> Matrix Multiply6/2
  Matrix Multiply6/1 -> Out1/1
  Constant2/1 -> Subsystem1/2(In2)

== system VFA_ActModel2_2015a/Adaptive Control/FL_Calculation/Filter2/Filter1 ==
  u1 : Inport
  u1dot : Inport  Port=2
  u1ddot : Inport  Port=3
  u2 : Inport  Port=4
  u2dot : Inport  Port=5
  u2ddot : Inport  Port=6
  Gain1 : Gain  Gain=d21
  Gain2 : Gain  Gain=d20
  Gain3 : Gain  Gain=d22
  Gain4 : Gain  Gain=a22
  Gain5 : Gain  Gain=d11
  Gain6 : Gain  Gain=d10
  Gain7 : Gain  Gain=a21
  Gain8 : Gain  Gain=d00
  Gain9 : Gain  Gain=a20
  Matrix Multiply{1..6} (6 alike) : Product  Multiplication=Matrix(*)
  Sum1 : Sum  Inputs=+++|
  Sum2 : Sum  Inputs=+++|
  Sum3 : Sum  Inputs=++|
  Out1 : Outport
  wires:
  u1/1 -> Matrix Multiply2/1, Matrix Multiply6/1, Matrix Multiply5/1
  u2ddot/1 -> Matrix Multiply2/2
  Matrix Multiply2/1 -> Gain2/1
  u1ddot/1 -> Matrix Multiply1/1
  u2/1 -> Matrix Multiply6/2, Matrix Multiply4/2, Matrix Multiply1/2
  Matrix Multiply1/1 -> Gain3/1
  u2dot/1 -> Matrix Multiply5/2, Matrix Multiply3/2
  u1dot/1 -> Matrix Multiply4/1, Matrix Multiply3/1
  Matrix Multiply3/1 -> Gain1/1
  Gain1/1 -> Sum1/3
  Gain3/1 -> Sum1/2
  Gain2/1 -> Sum1/1
  Sum1/1 -> Gain4/1
  Gain4/1 -> Sum2/1
  Matrix Multiply4/1 -> Gain5/1
  Gain5/1 -> Sum3/1
  Matrix Multiply5/1 -> Gain6/1
  Gain6/1 -> Sum3/2
  Sum3/1 -> Gain7/1
  Gain7/1 -> Sum2/2
  Matrix Multiply6/1 -> Gain8/1
  Gain8/1 -> Gain9/1
  Sum2/1 -> Out1/1
  Gain9/1 -> Sum2/3

== system VFA_ActModel2_2015a/Adaptive Control/FL_Calculation/Filter3/Ba3_aug Interpolation ==
  State : Inport
  eta : Inport  Port=2
  Constant2 : Constant  Value=Ba3_aug_M
  Gain : Gain  Gain=180/pi
  Matrix Multiply6 : Product  Multiplication=Matrix(*)
  Subsystem1 : Subsystem
      mask Display: disp('matrix-interp');
  Out1 : Outport
  wires:
  eta/1 -> Gain/1
  Gain/1 -> Subsystem1/1(In1)
  Subsystem1/1(Out1) -> Matrix Multiply6/1
  State/1 -> Matrix Multiply6/2
  Matrix Multiply6/1 -> Out1/1
  Constant2/1 -> Subsystem1/2(In2)

== system VFA_ActModel2_2015a/Adaptive Control/FL_Calculation/Filter3/Filter1 ==
  u1 : Inport
  u1dot : Inport  Port=2
  u1ddot : Inport  Port=3
  u2 : Inport  Port=4
  u2dot : Inport  Port=5
  u2ddot : Inport  Port=6
  Gain1 : Gain  Gain=d21
  Gain2 : Gain  Gain=d20
  Gain3 : Gain  Gain=d22
  Gain4 : Gain  Gain=a22
  Gain5 : Gain  Gain=d11
  Gain6 : Gain  Gain=d10
  Gain7 : Gain  Gain=a21
  Gain8 : Gain  Gain=d00
  Gain9 : Gain  Gain=a20
  Matrix Multiply{1..6} (6 alike) : Product  Multiplication=Matrix(*)
  Sum1 : Sum  Inputs=+++|
  Sum2 : Sum  Inputs=+++|
  Sum3 : Sum  Inputs=++|
  Out1 : Outport
  wires:
  u1/1 -> Matrix Multiply2/1, Matrix Multiply6/1, Matrix Multiply5/1
  u2ddot/1 -> Matrix Multiply2/2
  Matrix Multiply2/1 -> Gain2/1
  u1ddot/1 -> Matrix Multiply1/1
  u2/1 -> Matrix Multiply6/2, Matrix Multiply4/2, Matrix Multiply1/2
  Matrix Multiply1/1 -> Gain3/1
  u2dot/1 -> Matrix Multiply5/2, Matrix Multiply3/2
  u1dot/1 -> Matrix Multiply4/1, Matrix Multiply3/1
  Matrix Multiply3/1 -> Gain1/1
  Gain1/1 -> Sum1/3
  Gain3/1 -> Sum1/2
  Gain2/1 -> Sum1/1
  Sum1/1 -> Gain4/1
  Gain4/1 -> Sum2/1
  Matrix Multiply4/1 -> Gain5/1
  Gain5/1 -> Sum3/1
  Matrix Multiply5/1 -> Gain6/1
  Gain6/1 -> Sum3/2
  Sum3/1 -> Gain7/1
  Gain7/1 -> Sum2/2
  Matrix Multiply6/1 -> Gain8/1
  Gain8/1 -> Gain9/1
  Sum2/1 -> Out1/1
  Gain9/1 -> Sum2/3

== system VFA_ActModel2_2015a/Adaptive Control/FL_Calculation/Filter4/Subsystem ==
  In1 : Inport
  mu_psi : Inport  Port=2
  Constant : Constant
  Math Function1 : Math  Operator=transpose  SaturateOnIntegerOverflow=on
  Matrix Multiply6 : Product  Inputs=3  Multiplication=Matrix(*)
  Sum : Sum  Inputs=|++
  Out1 : Outport
  wires:
  In1/1 -> Matrix Multiply6/2, Math Function1/1
  Math Function1/1 -> Matrix Multiply6/1
  Constant/1 -> Sum/2
  Sum/1 -> Out1/1
  Matrix Multiply6/1 -> Sum/1
  mu_psi/1 -> Matrix Multiply6/3

== system VFA_ActModel2_2015a/Adaptive Control/FL_Calculation/Filter6/Subsystem ==
  In1 : Inport
  mu_psi : Inport  Port=2
  Constant : Constant
  Math Function1 : Math  Operator=transpose  SaturateOnIntegerOverflow=on
  Matrix Multiply6 : Product  Inputs=3  Multiplication=Matrix(*)
  Sum : Sum  Inputs=|++
  Out1 : Outport
  wires:
  In1/1 -> Matrix Multiply6/2, Math Function1/1
  Math Function1/1 -> Matrix Multiply6/1
  Constant/1 -> Sum/2
  Sum/1 -> Out1/1
  Matrix Multiply6/1 -> Sum/1
  mu_psi/1 -> Matrix Multiply6/3

== system VFA_ActModel2_2015a/Adaptive Control/Fxm_Calculation/Filter1/Ba3 Interpolation ==
  State : Inport
  eta : Inport  Port=2
  Constant2 : Constant  Value=Ba3_M
  Gain : Gain  Gain=180/pi
  Matrix Multiply6 : Product  Multiplication=Matrix(*)
  Subsystem1 : Subsystem
      mask Display: disp('matrix-interp');
  Out1 : Outport
  wires:
  eta/1 -> Gain/1
  Gain/1 -> Subsystem1/1(In1)
  Subsystem1/1(Out1) -> Matrix Multiply6/1
  State/1 -> Matrix Multiply6/2
  Matrix Multiply6/1 -> Out1/1
  Constant2/1 -> Subsystem1/2(In2)

== system VFA_ActModel2_2015a/Adaptive Control/Fxm_Calculation/Filter1/Ba32 Interpolation ==
  State : Inport
  eta : Inport  Port=2
  Constant2 : Constant  Value=Ba32_M
  Gain : Gain  Gain=180/pi
  Matrix Multiply6 : Product  Multiplication=Matrix(*)
  Subsystem1 : Subsystem
      mask Display: disp('matrix-interp');
  Out1 : Outport
  wires:
  eta/1 -> Gain/1
  Gain/1 -> Subsystem1/1(In1)
  Subsystem1/1(Out1) -> Matrix Multiply6/1
  State/1 -> Matrix Multiply6/2
  Matrix Multiply6/1 -> Out1/1
  Constant2/1 -> Subsystem1/2(In2)

== system VFA_ActModel2_2015a/Adaptive Control/Fxm_Calculation/Filter1/Filter15 ==
  u1 : Inport
  u1dot : Inport  Port=2
  u2 : Inport  Port=3
  u2dot : Inport  Port=4
  Gain2 : Gain  Gain=d10
  Gain25 : Gain  Gain=d11
  Matrix Multiply2 : Product  Multiplication=Matrix(*)
  Matrix Multiply3 : Product  Multiplication=Matrix(*)
  Sum2 : Sum  Inputs=++|
  Out1 : Outport
  wires:
  Matrix Multiply2/1 -> Gain2/1
  Matrix Multiply3/1 -> Gain25/1
  Gain25/1 -> Sum2/1
  u1dot/1 -> Matrix Multiply3/1
  u2/1 -> Matrix Multiply3/2
  u1/1 -> Matrix Multiply2/1
  u2dot/1 -> Matrix Multiply2/2
  Gain2/1 -> Sum2/2
  Sum2/1 -> Out1/1

== system VFA_ActModel2_2015a/Adaptive Control/Fxm_Calculation/Filter3/Ba3 Interpolation ==
  State : Inport
  eta : Inport  Port=2
  Constant2 : Constant  Value=Ba3_M
  Gain : Gain  Gain=180/pi
  Matrix Multiply6 : Product  Multiplication=Matrix(*)
  Subsystem1 : Subsystem
      mask Display: disp('matrix-interp');
  Out1 : Outport
  wires:
  eta/1 -> Gain/1
  Gain/1 -> Subsystem1/1(In1)
  Subsystem1/1(Out1) -> Matrix Multiply6/1
  State/1 -> Matrix Multiply6/2
  Matrix Multiply6/1 -> Out1/1
  Constant2/1 -> Subsystem1/2(In2)

== system VFA_ActModel2_2015a/Adaptive Control/Fxm_Calculation/Filter3/Filter1 ==
  u1 : Inport
  u1dot : Inport  Port=2
  u1ddot : Inport  Port=3
  u2 : Inport  Port=4
  u2dot : Inport  Port=5
  u2ddot : Inport  Port=6
  Gain1 : Gain  Gain=d21
  Gain2 : Gain  Gain=d20
  Gain3 : Gain  Gain=d22
  Gain4 : Gain  Gain=a22
  Gain5 : Gain  Gain=d11
  Gain6 : Gain  Gain=d10
  Gain7 : Gain  Gain=a21
  Gain8 : Gain  Gain=d00
  Gain9 : Gain  Gain=a20
  Matrix Multiply{1..6} (6 alike) : Product  Multiplication=Matrix(*)
  Sum1 : Sum  Inputs=+++|
  Sum2 : Sum  Inputs=+++|
  Sum3 : Sum  Inputs=++|
  Out1 : Outport
  wires:
  u1/1 -> Matrix Multiply2/1, Matrix Multiply6/1, Matrix Multiply5/1
  u2ddot/1 -> Matrix Multiply2/2
  Matrix Multiply2/1 -> Gain2/1
  u1ddot/1 -> Matrix Multiply1/1
  u2/1 -> Matrix Multiply6/2, Matrix Multiply4/2, Matrix Multiply1/2
  Matrix Multiply1/1 -> Gain3/1
  u2dot/1 -> Matrix Multiply5/2, Matrix Multiply3/2
  u1dot/1 -> Matrix Multiply4/1, Matrix Multiply3/1
  Matrix Multiply3/1 -> Gain1/1
  Gain1/1 -> Sum1/3
  Gain3/1 -> Sum1/2
  Gain2/1 -> Sum1/1
  Sum1/1 -> Gain4/1
  Gain4/1 -> Sum2/1
  Matrix Multiply4/1 -> Gain5/1
  Gain5/1 -> Sum3/1
  Matrix Multiply5/1 -> Gain6/1
  Gain6/1 -> Sum3/2
  Sum3/1 -> Gain7/1
  Gain7/1 -> Sum2/2
  Matrix Multiply6/1 -> Gain8/1
  Gain8/1 -> Gain9/1
  Sum2/1 -> Out1/1
  Gain9/1 -> Sum2/3

== system VFA_ActModel2_2015a/Adaptive Control/Fxm_Calculation/Filter5/Subsystem ==
  In1 : Inport
  mu_psi : Inport  Port=2
  Constant : Constant
  Math Function1 : Math  Operator=transpose  SaturateOnIntegerOverflow=on
  Matrix Multiply6 : Product  Inputs=3  Multiplication=Matrix(*)
  Sum : Sum  Inputs=|++
  Out1 : Outport
  wires:
  In1/1 -> Matrix Multiply6/2, Math Function1/1
  Math Function1/1 -> Matrix Multiply6/1
  Constant/1 -> Sum/2
  Sum/1 -> Out1/1
  Matrix Multiply6/1 -> Sum/1
  mu_psi/1 -> Matrix Multiply6/3

== system VFA_ActModel2_2015a/Adaptive Control/uad_Calculation/Filter10/Subsystem ==
  In1 : Inport
  mu_psi : Inport  Port=2
  Constant : Constant
  Math Function1 : Math  Operator=transpose  SaturateOnIntegerOverflow=on
  Matrix Multiply6 : Product  Inputs=3  Multiplication=Matrix(*)
  Sum : Sum  Inputs=|++
  Out1 : Outport
  wires:
  In1/1 -> Matrix Multiply6/2, Math Function1/1
  Math Function1/1 -> Matrix Multiply6/1
  Constant/1 -> Sum/2
  Sum/1 -> Out1/1
  Matrix Multiply6/1 -> Sum/1
  mu_psi/1 -> Matrix Multiply6/3

== system VFA_ActModel2_2015a/Adaptive Control/uad_Calculation/Filter12/Subsystem ==
  In1 : Inport
  mu_psi : Inport  Port=2
  Constant : Constant
  Math Function1 : Math  Operator=transpose  SaturateOnIntegerOverflow=on
  Matrix Multiply6 : Product  Inputs=3  Multiplication=Matrix(*)
  Sum : Sum  Inputs=|++
  Out1 : Outport
  wires:
  In1/1 -> Matrix Multiply6/2, Math Function1/1
  Math Function1/1 -> Matrix Multiply6/1
  Constant/1 -> Sum/2
  Sum/1 -> Out1/1
  Matrix Multiply6/1 -> Sum/1
  mu_psi/1 -> Matrix Multiply6/3

== system VFA_ActModel2_2015a/Adaptive Control/uad_Calculation/Filter7/Subsystem ==
  In1 : Inport
  mu_psi : Inport  Port=2
  Constant : Constant
  Math Function1 : Math  Operator=transpose  SaturateOnIntegerOverflow=on
  Matrix Multiply6 : Product  Inputs=3  Multiplication=Matrix(*)
  Sum : Sum  Inputs=|++
  Out1 : Outport
  wires:
  In1/1 -> Matrix Multiply6/2, Math Function1/1
  Math Function1/1 -> Matrix Multiply6/1
  Constant/1 -> Sum/2
  Sum/1 -> Out1/1
  Matrix Multiply6/1 -> Sum/1
  mu_psi/1 -> Matrix Multiply6/3

== system VFA_ActModel2_2015a/Adaptive Control/uad_Calculation/Filter9/Subsystem ==
  In1 : Inport
  mu_psi : Inport  Port=2
  Constant : Constant
  Math Function1 : Math  Operator=transpose  SaturateOnIntegerOverflow=on
  Matrix Multiply6 : Product  Inputs=3  Multiplication=Matrix(*)
  Sum : Sum  Inputs=|++
  Out1 : Outport
  wires:
  In1/1 -> Matrix Multiply6/2, Math Function1/1
  Math Function1/1 -> Matrix Multiply6/1
  Constant/1 -> Sum/2
  Sum/1 -> Out1/1
  Matrix Multiply6/1 -> Sum/1
  mu_psi/1 -> Matrix Multiply6/3

== system VFA_ActModel2_2015a/Adaptive Control/FL_Calculation/Filter1/Ba32_aug Interpolation/Subsystem1 ==
  In1 : Inport
  In2 : Inport  Port=2
  Bias1 : Bias  Bias=1
  Direct Lookup Table (n-D)2 : LookupNDDirect  NumberOfTableDimensions=3  InputsSelectThisObjectFromTable=2-D Matrix  TableIsInput=on  Table=ahold
  Direct Lookup Table (n-D)3 : LookupNDDirect  NumberOfTableDimensions=3  InputsSelectThisObjectFromTable=2-D Matrix  TableIsInput=on  Table=ahold
  Fcn1 : Fcn  Expr=1-u(1)
  Prelookup1 : PreLookup  BreakpointsData=etasweep  ExtrapMethod=Linear
  Product2 : Product  RndMeth=Zero
  Product3 : Product  RndMeth=Zero
  Sum1 : Sum  Inputs=|++
  Out1 : Outport
  wires:
  In1/1 -> Prelookup1/1
  Sum1/1 -> Out1/1
  Prelookup1/1 -> Direct Lookup Table (n-D)3/1, Bias1/1
  Direct Lookup Table (n-D)2/1 -> Product2/1
  Prelookup1/2 -> Product2/2, Fcn1/1
  Direct Lookup Table (n-D)3/1 -> Product3/1
  Product2/1 -> Sum1/1
  Product3/1 -> Sum1/2
  Bias1/1 -> Direct Lookup Table (n-D)2/1
  In2/1 -> Direct Lookup Table (n-D)3/2, Direct Lookup Table (n-D)2/2
  Fcn1/1 -> Product3/2

== system VFA_ActModel2_2015a/Adaptive Control/FL_Calculation/Filter1/Ba3_aug Interpolation/Subsystem1 ==
  In1 : Inport
  In2 : Inport  Port=2
  Bias1 : Bias  Bias=1
  Direct Lookup Table (n-D)2 : LookupNDDirect  NumberOfTableDimensions=3  InputsSelectThisObjectFromTable=2-D Matrix  TableIsInput=on  Table=ahold
  Direct Lookup Table (n-D)3 : LookupNDDirect  NumberOfTableDimensions=3  InputsSelectThisObjectFromTable=2-D Matrix  TableIsInput=on  Table=ahold
  Fcn1 : Fcn  Expr=1-u(1)
  Prelookup1 : PreLookup  BreakpointsData=etasweep  ExtrapMethod=Linear
  Product2 : Product  RndMeth=Zero
  Product3 : Product  RndMeth=Zero
  Sum1 : Sum  Inputs=|++
  Out1 : Outport
  wires:
  In1/1 -> Prelookup1/1
  Sum1/1 -> Out1/1
  Prelookup1/1 -> Direct Lookup Table (n-D)3/1, Bias1/1
  Direct Lookup Table (n-D)2/1 -> Product2/1
  Prelookup1/2 -> Product2/2, Fcn1/1
  Direct Lookup Table (n-D)3/1 -> Product3/1
  Product2/1 -> Sum1/1
  Product3/1 -> Sum1/2
  Bias1/1 -> Direct Lookup Table (n-D)2/1
  In2/1 -> Direct Lookup Table (n-D)3/2, Direct Lookup Table (n-D)2/2
  Fcn1/1 -> Product3/2

== system VFA_ActModel2_2015a/Adaptive Control/FL_Calculation/Filter2/Ba3_aug Interpolation/Subsystem1 ==
  In1 : Inport
  In2 : Inport  Port=2
  Bias1 : Bias  Bias=1
  Direct Lookup Table (n-D)2 : LookupNDDirect  NumberOfTableDimensions=3  InputsSelectThisObjectFromTable=2-D Matrix  TableIsInput=on  Table=ahold
  Direct Lookup Table (n-D)3 : LookupNDDirect  NumberOfTableDimensions=3  InputsSelectThisObjectFromTable=2-D Matrix  TableIsInput=on  Table=ahold
  Fcn1 : Fcn  Expr=1-u(1)
  Prelookup1 : PreLookup  BreakpointsData=etasweep  ExtrapMethod=Linear
  Product2 : Product  RndMeth=Zero
  Product3 : Product  RndMeth=Zero
  Sum1 : Sum  Inputs=|++
  Out1 : Outport
  wires:
  In1/1 -> Prelookup1/1
  Sum1/1 -> Out1/1
  Prelookup1/1 -> Direct Lookup Table (n-D)3/1, Bias1/1
  Direct Lookup Table (n-D)2/1 -> Product2/1
  Prelookup1/2 -> Product2/2, Fcn1/1
  Direct Lookup Table (n-D)3/1 -> Product3/1
  Product2/1 -> Sum1/1
  Product3/1 -> Sum1/2
  Bias1/1 -> Direct Lookup Table (n-D)2/1
  In2/1 -> Direct Lookup Table (n-D)3/2, Direct Lookup Table (n-D)2/2
  Fcn1/1 -> Product3/2

== system VFA_ActModel2_2015a/Adaptive Control/FL_Calculation/Filter3/Ba3_aug Interpolation/Subsystem1 ==
  In1 : Inport
  In2 : Inport  Port=2
  Bias1 : Bias  Bias=1
  Direct Lookup Table (n-D)2 : LookupNDDirect  NumberOfTableDimensions=3  InputsSelectThisObjectFromTable=2-D Matrix  TableIsInput=on  Table=ahold
  Direct Lookup Table (n-D)3 : LookupNDDirect  NumberOfTableDimensions=3  InputsSelectThisObjectFromTable=2-D Matrix  TableIsInput=on  Table=ahold
  Fcn1 : Fcn  Expr=1-u(1)
  Prelookup1 : PreLookup  BreakpointsData=etasweep  ExtrapMethod=Linear
  Product2 : Product  RndMeth=Zero
  Product3 : Product  RndMeth=Zero
  Sum1 : Sum  Inputs=|++
  Out1 : Outport
  wires:
  In1/1 -> Prelookup1/1
  Sum1/1 -> Out1/1
  Prelookup1/1 -> Direct Lookup Table (n-D)3/1, Bias1/1
  Direct Lookup Table (n-D)2/1 -> Product2/1
  Prelookup1/2 -> Product2/2, Fcn1/1
  Direct Lookup Table (n-D)3/1 -> Product3/1
  Product2/1 -> Sum1/1
  Product3/1 -> Sum1/2
  Bias1/1 -> Direct Lookup Table (n-D)2/1
  In2/1 -> Direct Lookup Table (n-D)3/2, Direct Lookup Table (n-D)2/2
  Fcn1/1 -> Product3/2

== system VFA_ActModel2_2015a/Adaptive Control/Fxm_Calculation/Filter1/Ba3 Interpolation/Subsystem1 ==
  In1 : Inport
  In2 : Inport  Port=2
  Bias1 : Bias  Bias=1
  Direct Lookup Table (n-D)2 : LookupNDDirect  NumberOfTableDimensions=3  InputsSelectThisObjectFromTable=2-D Matrix  TableIsInput=on  Table=ahold
  Direct Lookup Table (n-D)3 : LookupNDDirect  NumberOfTableDimensions=3  InputsSelectThisObjectFromTable=2-D Matrix  TableIsInput=on  Table=ahold
  Fcn1 : Fcn  Expr=1-u(1)
  Prelookup1 : PreLookup  BreakpointsData=etasweep  ExtrapMethod=Linear
  Product2 : Product  RndMeth=Zero
  Product3 : Product  RndMeth=Zero
  Sum1 : Sum  Inputs=|++
  Out1 : Outport
  wires:
  In1/1 -> Prelookup1/1
  Sum1/1 -> Out1/1
  Prelookup1/1 -> Direct Lookup Table (n-D)3/1, Bias1/1
  Direct Lookup Table (n-D)2/1 -> Product2/1
  Prelookup1/2 -> Product2/2, Fcn1/1
  Direct Lookup Table (n-D)3/1 -> Product3/1
  Product2/1 -> Sum1/1
  Product3/1 -> Sum1/2
  Bias1/1 -> Direct Lookup Table (n-D)2/1
  In2/1 -> Direct Lookup Table (n-D)3/2, Direct Lookup Table (n-D)2/2
  Fcn1/1 -> Product3/2

== system VFA_ActModel2_2015a/Adaptive Control/Fxm_Calculation/Filter1/Ba32 Interpolation/Subsystem1 ==
  In1 : Inport
  In2 : Inport  Port=2
  Bias1 : Bias  Bias=1
  Direct Lookup Table (n-D)2 : LookupNDDirect  NumberOfTableDimensions=3  InputsSelectThisObjectFromTable=2-D Matrix  TableIsInput=on  Table=ahold
  Direct Lookup Table (n-D)3 : LookupNDDirect  NumberOfTableDimensions=3  InputsSelectThisObjectFromTable=2-D Matrix  TableIsInput=on  Table=ahold
  Fcn1 : Fcn  Expr=1-u(1)
  Prelookup1 : PreLookup  BreakpointsData=etasweep  ExtrapMethod=Linear
  Product2 : Product  RndMeth=Zero
  Product3 : Product  RndMeth=Zero
  Sum1 : Sum  Inputs=|++
  Out1 : Outport
  wires:
  In1/1 -> Prelookup1/1
  Sum1/1 -> Out1/1
  Prelookup1/1 -> Direct Lookup Table (n-D)3/1, Bias1/1
  Direct Lookup Table (n-D)2/1 -> Product2/1
  Prelookup1/2 -> Product2/2, Fcn1/1
  Direct Lookup Table (n-D)3/1 -> Product3/1
  Product2/1 -> Sum1/1
  Product3/1 -> Sum1/2
  Bias1/1 -> Direct Lookup Table (n-D)2/1
  In2/1 -> Direct Lookup Table (n-D)3/2, Direct Lookup Table (n-D)2/2
  Fcn1/1 -> Product3/2

== system VFA_ActModel2_2015a/Adaptive Control/Fxm_Calculation/Filter3/Ba3 Interpolation/Subsystem1 ==
  In1 : Inport
  In2 : Inport  Port=2
  Bias1 : Bias  Bias=1
  Direct Lookup Table (n-D)2 : LookupNDDirect  NumberOfTableDimensions=3  InputsSelectThisObjectFromTable=2-D Matrix  TableIsInput=on  Table=ahold
  Direct Lookup Table (n-D)3 : LookupNDDirect  NumberOfTableDimensions=3  InputsSelectThisObjectFromTable=2-D Matrix  TableIsInput=on  Table=ahold
  Fcn1 : Fcn  Expr=1-u(1)
  Prelookup1 : PreLookup  BreakpointsData=etasweep  ExtrapMethod=Linear
  Product2 : Product  RndMeth=Zero
  Product3 : Product  RndMeth=Zero
  Sum1 : Sum  Inputs=|++
  Out1 : Outport
  wires:
  In1/1 -> Prelookup1/1
  Sum1/1 -> Out1/1
  Prelookup1/1 -> Direct Lookup Table (n-D)3/1, Bias1/1
  Direct Lookup Table (n-D)2/1 -> Product2/1
  Prelookup1/2 -> Product2/2, Fcn1/1
  Direct Lookup Table (n-D)3/1 -> Product3/1
  Product2/1 -> Sum1/1
  Product3/1 -> Sum1/2
  Bias1/1 -> Direct Lookup Table (n-D)2/1
  In2/1 -> Direct Lookup Table (n-D)3/2, Direct Lookup Table (n-D)2/2
  Fcn1/1 -> Product3/2
